simulink model "CS6376_AircraftCollisionAvoidanceProject_RonaldPicard"  (R2018b)
settings: Solver=FixedStepAuto  StartTime=0.0  StopTime=10000  FixedStep=1  RelTol=1e-3
(part 2 of 2)

== stateflow chart CS6376_AircraftCollisionAvoidanceProject_RonaldPicard/Aircraft1/AircraftCollisionAvoidenceController ==
  settings: executeAtInitialization=1  initializeOutput=1
  state Controller
    du:
    Y_Out = Y_State;
    X_Out = X_State;
    Orientation_Out = Orientation_State;
    DangerZoneBreached_Out = 0;
    state CollisionAvoidanceMonitor90
      state InitTurn90_From0
        en:
        Orientation_State = 0;
        X_State = X_State + 1;
        Turning_State = Turning_State - 1;
      state AvoidCollisionTraveling0
        en:
        Orientation_State = 0;
        X_State = X_State + 1;
        Rounds_State = Rounds_State - 1;
        % initialize turn time
        Turning_State = Turning_Rounds_In;
      state InitTurn0
        en:
        Orientation_State = 90;
        Y_State = Y_State + 1;
        Rounds_State = Rounds_In;
        Turning_State = Turning_State - 1;
        % initialize rounds to avoid
        Rounds_State = Rounds_In;
      state Traveling90
        en:
        Orientation_State = 90;
        Y_State = Y_State + 1;
        % initialize turn time
        Turning_State = Turning_Rounds_In;
      state AvoidCollisionTraveling180
        en:
        Orientation_State = 180;
        X_State = X_State - 1;
        Rounds_State = Rounds_State - 1;
        % initialize turn time
        Turning_State = Turning_Rounds_In;
      state InitTurn180
        en:
        Orientation_State = 90;
        Y_State = Y_State + 1;
        Turning_State = Turning_State - 1;
        % initialize rounds to avoid
        Rounds_State = Rounds_In;
      state InitTurn90_From180
        en:
        Orientation_State = 180;
        X_State = X_State - 1;
        Turning_State = Turning_State - 1;
      (junction 582) -> InitTurn90_From0 : %else
      (junction 575) -> (junction 577) [order 2]
      (junction 575) -> InitTurn90_From0 [order 1] : % still turning
          | [Turning_State >0]
      (junction 305) -> (junction 582) [order 2]
      (junction 577) -> Traveling90
      (junction 581) -> (junction 575)
      (junction 305) -> Controller.CollisionAvoidanceMonitor90.AvoidCollisionTraveling0 [order 1] : % incoming aircraft quadrant 3 heading up or right
          | [Mess_Rec_In &&...
          | (X_Mess_In <= X_State) && (Y_Mess_In <= Y_State) &&...
          | (Orientation_Mess_In == 0 || Orientation_Mess_In == 90)]
      (junction 314) -> (junction 305) [order 2]
      InitTurn90_From0 -> (junction 581)
      (default) -> Traveling90
      (junction 314) -> Controller.CollisionAvoidanceMonitor90.AvoidCollisionTraveling0 [order 1] : % incoming aircraft quadrant 2 heading right or down
          | [Mess_Rec_In &&...
          | (X_Mess_In <= X_State) && (Y_Mess_In >= Y_State) &&...
          | (Orientation_Mess_In == 0 || Orientation_Mess_In == 270)]
      (junction 419) -> (junction 314) [order 2]
      (junction 298) -> Traveling90 [order 2] : %else
      (junction 298) -> Controller.CollisionAvoidanceMonitor90.InitTurn0 [order 1] : % incoming aircraft quadrant 3 heading up or right
          | [Mess_Rec_In &&...
          | (X_Mess_In <= X_State) && (Y_Mess_In <= Y_State) &&...
          | (Orientation_Mess_In == 0 || Orientation_Mess_In == 90)]
      (junction 308) -> (junction 298) [order 2]
      (junction 494) -> Controller.CollisionAvoidanceMonitor90.InitTurn0 [order 1] : % still turning
          | [Turning_State >0]
      (junction 494) -> Controller.CollisionAvoidanceMonitor90.AvoidCollisionTraveling0 [order 2]
      (junction 488) -> (junction 494)
      (junction 419) -> Controller.CollisionAvoidanceMonitor90.AvoidCollisionTraveling0 [order 1] : % still avoiding
          | [Rounds_State > 0]
      (junction 296) -> (junction 419)
      (junction 308) -> Controller.CollisionAvoidanceMonitor90.InitTurn0 [order 1] : % incoming aircraft quadrant 2 heading right or down
          | [Mess_Rec_In &&...
          | (X_Mess_In <= X_State) && (Y_Mess_In >= Y_State) &&...
          | (Orientation_Mess_In == 0 || Orientation_Mess_In == 270)]
      (junction 299) -> (junction 308) [order 2]
      Controller.CollisionAvoidanceMonitor90.AvoidCollisionTraveling0 -> (junction 296) : %each round
      Controller.CollisionAvoidanceMonitor90.InitTurn0 -> (junction 488) : %each round
      Controller.CollisionAvoidanceMonitor90.AvoidCollisionTraveling180 -> (junction 316) : %each round
      (junction 316) -> (junction 416)
      (junction 491) -> Controller.CollisionAvoidanceMonitor90.InitTurn180 [order 1] : % still turning
          | [Turning_State >0]
      (junction 491) -> Controller.CollisionAvoidanceMonitor90.AvoidCollisionTraveling180 [order 2]
      (junction 489) -> (junction 491)
      (junction 299) -> Controller.CollisionAvoidanceMonitor90.InitTurn180 [order 1] : % incoming aircraft quadrant 1 heading left or down
          | [Mess_Rec_In &&...
          | (X_Mess_In > X_State) && (Y_Mess_In >= Y_State) &&...
          | (Orientation_Mess_In == 180 || Orientation_Mess_In == 270)]
      (junction 309) -> (junction 299) [order 2]
      (junction 416) -> Controller.CollisionAvoidanceMonitor90.AvoidCollisionTraveling180 [order 1] : % still avoiding
          | [Rounds_State > 0]
      (junction 416) -> (junction 301) [order 2]
      Traveling90 -> (junction 309) : %each round
      (junction 309) -> Controller.CollisionAvoidanceMonitor90.InitTurn180 [order 1] : % incoming aircraft quadrant 4 heading up or left
          | [Mess_Rec_In &&...
          | (X_Mess_In > X_State) &&  (Y_Mess_In <= Y_State) &&...
          | (Orientation_Mess_In == 180 || Orientation_Mess_In == 90)]
      (junction 301) -> Controller.CollisionAvoidanceMonitor90.AvoidCollisionTraveling180 [order 1] : % incoming aircraft quadrant 1 heading left or down
          | [Mess_Rec_In &&...
          | (X_Mess_In > X_State) && (Y_Mess_In >= Y_State) &&...
          | (Orientation_Mess_In == 180 || Orientation_Mess_In == 270)]
      (junction 301) -> (junction 311) [order 2]
      Controller.CollisionAvoidanceMonitor90.InitTurn180 -> (junction 489) : %each round
      (junction 586) -> Traveling90
      (junction 311) -> Controller.CollisionAvoidanceMonitor90.AvoidCollisionTraveling180 [order 1] : % incoming aircraft quadrant 4 heading up or left
          | [Mess_Rec_In &&...
          | (X_Mess_In > X_State) &&  (Y_Mess_In <= Y_State) &&...
          | (Orientation_Mess_In == 180 || Orientation_Mess_In == 90)]
      (junction 311) -> (junction 594) [order 2]
      (junction 588) -> (junction 586) [order 2]
      (junction 588) -> InitTurn90_From180 [order 1] : % still turning
          | [Turning_State >0]
      (junction 587) -> (junction 588)
      (junction 594) -> InitTurn90_From180 : %else
      InitTurn90_From180 -> (junction 587)
    state Turn180_From90
      en:
      Orientation_State = 90;
      Y_State = Y_State + 1;
      Turning_State = Turning_State - 1;
    state Turn90_From0
      en:
      Orientation_State = 0;
      X_State = X_State + 1;
      Turning_State = Turning_State - 1;
    state Turn_90_From180
      en:
      Orientation_State = 180;
      X_State = X_State - 1;
      Turning_State = Turning_State - 1;
    state Turn90_From01
      en:
      Orientation_State = 90;
      Y_State = Y_State + 1;
      Turning_State = Turning_State - 1;
    state CollisionAvoidanceMonitor0
      state Turn0_From90
        en:
        Orientation_State = 90;
        Y_State = Y_State + 1;
        Turning_State = Turning_State - 1;
      state AvoidCollisionTraveling90
        en:
        Orientation_State = 90;
        Y_State = Y_State + 1;
        Rounds_State = Rounds_State - 1;
        % initialize turn time
        Turning_State = Turning_Rounds_In;
      state Turn90
        en:
        Orientation_State = 0;
        X_State = X_State + 1;
        Turning_State = Turning_State - 1;
        % initialize rounds to avoid
        Rounds_State = Rounds_In;
      state Traveling0
        en:
        Orientation_State = 0;
        X_State = X_State + 1;
        % initialize turn time
        Turning_State = Turning_Rounds_In;
      state Turn270
        en:
        Orientation_State = 0;
        X_State = X_State + 1;
        Turning_State = Turning_State - 1;
        % initialize rounds to avoid
        Rounds_State = Rounds_In;
      state AvoidCollisionTraveling270
        en:
        Orientation_State = 270;
        Y_State = Y_State - 1;
        Rounds_State = Rounds_State - 1;
        % initialize turn time
        Turning_State = Turning_Rounds_In;
      state Turn0_From270
        en:
        Orientation_State = 270;
        Y_State = Y_State - 1;
        Turning_State = Turning_State - 1;
      (junction 518) -> Turn0_From90 : %else
      (junction 227) -> (junction 518) [order 2]
      (junction 513) -> (junction 520) [order 2]
      (junction 513) -> Turn0_From90 [order 1] : % still turning
          | [Turning_State >0]
      (junction 520) -> Traveling0
      (junction 516) -> (junction 513)
      Turn0_From90 -> (junction 516)
      (junction 227) -> Controller.CollisionAvoidanceMonitor0.AvoidCollisionTraveling90 [order 1] : % incoming aircraft quadrant 3 heading up or right
          | [Mess_Rec_In &&...
          | (X_Mess_In <= X_State) && (Y_Mess_In <= Y_State) &&...
          | (Orientation_Mess_In == 0 || Orientation_Mess_In == 90)]
      (junction 219) -> (junction 227) [order 2]
      (default) -> Traveling0
      (junction 219) -> Controller.CollisionAvoidanceMonitor0.AvoidCollisionTraveling90 [order 1] : % incoming aircraft quadrant 4 heading up or left
          | [Mess_Rec_In &&...
          | (X_Mess_In >= X_State) && (Y_Mess_In <= Y_State) &&...
          | (Orientation_Mess_In == 180 || Orientation_Mess_In == 90)]
      (junction 381) -> (junction 219) [order 2]
      (junction 450) -> Turn90 [order 1] : % still turning
          | [Turning_State >0]
      (junction 450) -> Controller.CollisionAvoidanceMonitor0.AvoidCollisionTraveling90 [order 2]
      (junction 446) -> (junction 450)
      (junction 207) -> Traveling0 [order 2] : %else
      (junction 207) -> Turn90 [order 1] : % incoming aircraft quadrant 3 heading up or right
          | [Mess_Rec_In &&...
          | (X_Mess_In <= X_State) && (Y_Mess_In <= Y_State) &&...
          | (Orientation_Mess_In == 0 || Orientation_Mess_In == 90)]
      (junction 206) -> (junction 207) [order 2]
      (junction 381) -> Controller.CollisionAvoidanceMonitor0.AvoidCollisionTraveling90 [order 1] : % still avoiding
          | [Rounds_State > 0]
      (junction 220) -> (junction 381)
      Turn90 -> (junction 446) : %each round
      (junction 206) -> Turn90 [order 1] : % incoming aircraft quadrant 4 heading up or left
          | [Mess_Rec_In &&...
          | (X_Mess_In >= X_State) &&  (Y_Mess_In <= Y_State) &&...
          | (Orientation_Mess_In == 180 || Orientation_Mess_In == 90)]
      Controller.CollisionAvoidanceMonitor0.AvoidCollisionTraveling90 -> (junction 220) : %each round
      (junction 213) -> (junction 206) [order 2]
      Controller.CollisionAvoidanceMonitor0.AvoidCollisionTraveling270 -> (junction 230) : %each round
      (junction 213) -> Turn270 [order 1] : % incoming aircraft quadrant 1 heading left or down
          | [Mess_Rec_In &&...
          | (X_Mess_In >= X_State) && (Y_Mess_In > Y_State) &&...
          | (Orientation_Mess_In == 180 || Orientation_Mess_In == 270)]
      (junction 230) -> (junction 384)
      (junction 457) -> Controller.CollisionAvoidanceMonitor0.AvoidCollisionTraveling270 [order 2]
      (junction 457) -> Turn270 [order 1] : % still turning
          | [Turning_State >0]
      (junction 212) -> (junction 213) [order 2]
      (junction 455) -> (junction 457)
      (junction 384) -> Controller.CollisionAvoidanceMonitor0.AvoidCollisionTraveling270 [order 1] : % still avoiding
          | [Rounds_State > 0]
      (junction 384) -> (junction 240) [order 2]
      Traveling0 -> (junction 212) : %each round
      (junction 212) -> Turn270 [order 1] : % incoming aircraft quadrant 2 heading right or down
          | [Mess_Rec_In &&...
          | (X_Mess_In <= X_State) && (Y_Mess_In > Y_State) &&...
          | (Orientation_Mess_In == 0 || Orientation_Mess_In == 270)]
      (junction 240) -> Controller.CollisionAvoidanceMonitor0.AvoidCollisionTraveling270 [order 1] : % incoming aircraft quadrant 1 heading left or down
          | [Mess_Rec_In &&...
          | (X_Mess_In >= X_State) && (Y_Mess_In > Y_State) &&...
          | (Orientation_Mess_In == 180 || Orientation_Mess_In == 270)]
      Turn270 -> (junction 455) : %each round
      (junction 240) -> (junction 238) [order 2]
      (junction 508) -> Traveling0
      (junction 238) -> Controller.CollisionAvoidanceMonitor0.AvoidCollisionTraveling270 [order 1] : % incoming aircraft quadrant 2 heading right or down
          | [Mess_Rec_In &&...
          | (X_Mess_In <= X_State) && (Y_Mess_In > Y_State) &&...
          | (Orientation_Mess_In == 0 || Orientation_Mess_In == 270)]
      (junction 238) -> (junction 498) [order 2]
      (junction 504) -> (junction 508) [order 2]
      (junction 504) -> Controller.CollisionAvoidanceMonitor0.Turn0_From270 [order 1] : % still turning
          | [Turning_State >0]
      (junction 502) -> (junction 504)
      Controller.CollisionAvoidanceMonitor0.Turn0_From270 -> (junction 502)
      (junction 498) -> Controller.CollisionAvoidanceMonitor0.Turn0_From270 : %else
    state CollisionAvoidanceMonitor180
      state InitTurn180_From90
        en:
        Orientation_State = 90;
        Y_State = Y_State + 1;
        Turning_State = Turning_State - 1;
      state AvoidCollisionTraveling90
        en:
        Orientation_State = 90;
        Y_State = Y_State + 1;
        Rounds_State = Rounds_State - 1;
        % initialize turn time
        Turning_State = Turning_Rounds_In;
      state Traveling180
        en:
        Orientation_State = 180;
        X_State = X_State - 1;
        % initialize turn time
        Turning_State = Turning_Rounds_In;
      state InitTurn90
        en:
        Orientation_State = 180;
        X_State = X_State - 1;
        Turning_State = Turning_State - 1;
        % initialize rounds to avoid
        Rounds_State = Rounds_In;
      state AvoidCollisionTraveling270
        en:
        Orientation_State = 270;
        Y_State = Y_State - 1;
        Rounds_State = Rounds_State - 1;
        % initialize turn time
        Turning_State = Turning_Rounds_In;
      state InitTurn270
        en:
        Orientation_State = 180;
        X_State = X_State - 1;
        Turning_State = Turning_State - 1;
        % initialize rounds to avoid
        Rounds_State = Rounds_In;
      state InitTurn180_From270
        en:
        Orientation_State = 270;
        Y_State = Y_State - 1;
        Turning_State = Turning_State - 1;
      (junction 544) -> InitTurn180_From90 : %else
      (junction 286) -> (junction 544) [order 2]
      (junction 538) -> (junction 543) [order 2]
      (junction 538) -> InitTurn180_From90 [order 1] : % still turning
          | [Turning_State >0]
      (junction 543) -> Traveling180
      (junction 540) -> (junction 538)
      (junction 286) -> Controller.CollisionAvoidanceMonitor180.AvoidCollisionTraveling90 [order 1] : % incoming aircraft quadrant 3 heading up or right
          | [Mess_Rec_In &&...
          | (X_Mess_In <= X_State) && (Y_Mess_In < Y_State) &&...
          | (Orientation_Mess_In == 0 || Orientation_Mess_In == 90)]
      InitTurn180_From90 -> (junction 540)
      (junction 269) -> (junction 286) [order 2]
      (default) -> Traveling180
      (junction 269) -> Controller.CollisionAvoidanceMonitor180.AvoidCollisionTraveling90 [order 1] : % incoming aircraft quadrant 4 heading up or left
          | [Mess_Rec_In &&...
          | (X_Mess_In >= X_State) && (Y_Mess_In < Y_State) &&...
          | (Orientation_Mess_In == 180 || Orientation_Mess_In == 90)]
      (junction 406) -> (junction 269) [order 2]
      (junction 279) -> InitTurn90 [order 1] : % incoming aircraft quadrant 3 heading up or right
          | [Mess_Rec_In &&...
          | (X_Mess_In <= X_State) && (Y_Mess_In < Y_State) &&...
          | (Orientation_Mess_In == 0 || Orientation_Mess_In == 90)]
      (junction 279) -> Traveling180 [order 2] : %else
      (junction 483) -> InitTurn90 [order 1] : % still turning
          | [Turning_State >0]
      (junction 483) -> Controller.CollisionAvoidanceMonitor180.AvoidCollisionTraveling90 [order 2]
      (junction 287) -> (junction 279) [order 2]
      (junction 479) -> (junction 483)
      (junction 406) -> Controller.CollisionAvoidanceMonitor180.AvoidCollisionTraveling90 [order 1] : % still avoiding
          | [Rounds_State > 0]
      (junction 288) -> (junction 406)
      (junction 287) -> InitTurn90 [order 1] : % incoming aircraft quadrant 4 heading up or left
          | [Mess_Rec_In &&...
          | (X_Mess_In >= X_State) &&  (Y_Mess_In < Y_State) &&...
          | (Orientation_Mess_In == 180 || Orientation_Mess_In == 90)]
      (junction 276) -> (junction 287) [order 2]
      InitTurn90 -> (junction 479) : %each round
      Controller.CollisionAvoidanceMonitor180.AvoidCollisionTraveling90 -> (junction 288) : %each round
      (junction 481) -> Controller.CollisionAvoidanceMonitor180.AvoidCollisionTraveling270 [order 2]
      (junction 481) -> InitTurn270 [order 1] : % still turning
          | [Turning_State >0]
      (junction 276) -> InitTurn270 [order 1] : % incoming aircraft quadrant 1 heading left or down
          | [Mess_Rec_In &&...
          | (X_Mess_In >= X_State) && (Y_Mess_In >= Y_State) &&...
          | (Orientation_Mess_In == 180 || Orientation_Mess_In == 270)]
      Controller.CollisionAvoidanceMonitor180.AvoidCollisionTraveling270 -> (junction 270) : %each round
      (junction 475) -> (junction 481)
      (junction 271) -> (junction 276) [order 2]
      (junction 270) -> (junction 404)
      Traveling180 -> (junction 271) : %each round
      (junction 271) -> InitTurn270 [order 1] : % incoming aircraft quadrant 2 heading right or down
          | [Mess_Rec_In &&...
          | (X_Mess_In <= X_State) && (Y_Mess_In >= Y_State) &&...
          | (Orientation_Mess_In == 0 || Orientation_Mess_In == 270)]
      (junction 404) -> Controller.CollisionAvoidanceMonitor180.AvoidCollisionTraveling270 [order 1] : % still avoiding
          | [Rounds_State > 0]
      (junction 404) -> (junction 289) [order 2]
      InitTurn270 -> (junction 475) : %each round
      (junction 289) -> Controller.CollisionAvoidanceMonitor180.AvoidCollisionTraveling270 [order 1] : % incoming aircraft quadrant 1 heading left or down
          | [Mess_Rec_In &&...
          | (X_Mess_In >= X_State) && (Y_Mess_In >= Y_State) &&...
          | (Orientation_Mess_In == 180 || Orientation_Mess_In == 270)]
      (junction 289) -> (junction 272) [order 2]
      (junction 526) -> Traveling180
      (junction 272) -> Controller.CollisionAvoidanceMonitor180.AvoidCollisionTraveling270 [order 1] : % incoming aircraft quadrant 2 heading right or down
          | [Mess_Rec_In &&...
          | (X_Mess_In <= X_State) && (Y_Mess_In >= Y_State) &&...
          | (Orientation_Mess_In == 0 || Orientation_Mess_In == 270)]
      (junction 272) -> (junction 532) [order 2]
      (junction 525) -> (junction 526) [order 2]
      (junction 525) -> InitTurn180_From270 [order 1] : % still turning
          | [Turning_State >0]
      (junction 530) -> (junction 525)
      InitTurn180_From270 -> (junction 530)
      (junction 532) -> InitTurn180_From270 : %else
    state Initialize
      en:
      X_State = Initial_X;
      Y_State = Initial_Y;
      Orientation_State = Initial_Orientation;
    state CollisionAvoidanceMonitor270
      state InitTurn270_From0
        en:
        Orientation_State = 0;
        X_State = X_State + 1;
        Turning_State = Turning_State - 1;
      state AvoidCollisionTraveling0
        en:
        Orientation_State = 0;
        X_State = X_State + 1;
        Rounds_State = Rounds_State - 1;
        % initialize turn time
        Turning_State = Turning_Rounds_In;
      state InitTurn0
        en:
        Orientation_State = 270;
        Y_State = Y_State - 1
        Turning_State = Turning_State - 1;
        % initialize rounds to avoid
        Rounds_State = Rounds_In;
      state Traveling270
        en:
        Orientation_State = 270;
        Y_State = Y_State - 1
        % initialize turn time
        Turning_State = Turning_Rounds_In;
      state InitTurn180
        en:
        Orientation_State = 270;
        Y_State = Y_State - 1
        Turning_State = Turning_State - 1;
        % initialize rounds to avoid
        Rounds_State = Rounds_In;
      state AvoidCollisionTraveling180
        en:
        Orientation_State = 180;
        X_State = X_State - 1;
        Rounds_State = Rounds_State - 1;
        % initialize turn time
        Turning_State = Turning_Rounds_In;
      state InitTurn270_From180
        en:
        Orientation_State = 180;
        X_State = X_State - 1;
        Turning_State = Turning_State - 1;
      (junction 569) -> InitTurn270_From0 : %else
      (junction 563) -> (junction 565) [order 2]
      (junction 563) -> InitTurn270_From0 [order 1] : % still turning
          | [Turning_State >0]
      (junction 338) -> (junction 569) [order 2]
      (junction 565) -> Traveling270
      (junction 568) -> (junction 563)
      InitTurn270_From0 -> (junction 568)
      (junction 338) -> Controller.CollisionAvoidanceMonitor270.AvoidCollisionTraveling0 [order 1] : % incoming aircraft quadrant 3 heading up or right
          | [Mess_Rec_In &&...
          | (X_Mess_In < X_State) && (Y_Mess_In <= Y_State) &&...
          | (Orientation_Mess_In == 0 || Orientation_Mess_In == 90)]
      (junction 354) -> (junction 338) [order 2]
      (default) -> Traveling270
      (junction 354) -> Controller.CollisionAvoidanceMonitor270.AvoidCollisionTraveling0 [order 1] : % incoming aircraft quadrant 2 heading right or down
          | [Mess_Rec_In &&...
          | (X_Mess_In < X_State) && (Y_Mess_In >= Y_State) &&...
          | (Orientation_Mess_In == 0 || Orientation_Mess_In == 270)]
      (junction 394) -> (junction 354) [order 2]
      (junction 466) -> Controller.CollisionAvoidanceMonitor270.AvoidCollisionTraveling0 [order 2]
      (junction 466) -> Controller.CollisionAvoidanceMonitor270.InitTurn0 [order 1] : % still turning
          | [Turning_State >0]
      (junction 460) -> (junction 466)
      (junction 333) -> Controller.CollisionAvoidanceMonitor270.InitTurn0 [order 1] : % incoming aircraft quadrant 3 heading up or right
          | [Mess_Rec_In &&...
          | (X_Mess_In < X_State) && (Y_Mess_In <= Y_State) &&...
          | (Orientation_Mess_In == 0 || Orientation_Mess_In == 90)]
      (junction 333) -> Traveling270 [order 2] : %else
      (junction 357) -> (junction 333) [order 2]
      (junction 394) -> Controller.CollisionAvoidanceMonitor270.AvoidCollisionTraveling0 [order 1] : % still avoiding
          | [Rounds_State > 0]
      (junction 337) -> (junction 394)
      (junction 357) -> Controller.CollisionAvoidanceMonitor270.InitTurn0 [order 1] : % incoming aircraft quadrant 2 heading right or down
          | [Mess_Rec_In &&...
          | (X_Mess_In < X_State) && (Y_Mess_In >= Y_State) &&...
          | (Orientation_Mess_In == 0 || Orientation_Mess_In == 270)]
      Controller.CollisionAvoidanceMonitor270.InitTurn0 -> (junction 460) : %each round
      (junction 334) -> (junction 357) [order 2]
      Controller.CollisionAvoidanceMonitor270.AvoidCollisionTraveling0 -> (junction 337) : %each round
      (junction 464) -> Controller.CollisionAvoidanceMonitor270.InitTurn180 [order 1] : % still turning
          | [Turning_State >0]
      (junction 464) -> Controller.CollisionAvoidanceMonitor270.AvoidCollisionTraveling180 [order 2]
      Controller.CollisionAvoidanceMonitor270.AvoidCollisionTraveling180 -> (junction 361) : %each round
      (junction 469) -> (junction 464)
      (junction 361) -> (junction 397)
      (junction 334) -> Controller.CollisionAvoidanceMonitor270.InitTurn180 [order 1] : % incoming aircraft quadrant 1 heading left or down
          | [Mess_Rec_In &&...
          | (X_Mess_In >= X_State) && (Y_Mess_In >= Y_State) &&...
          | (Orientation_Mess_In == 180 || Orientation_Mess_In == 270)]
      (junction 347) -> (junction 334) [order 2]
      (junction 397) -> Controller.CollisionAvoidanceMonitor270.AvoidCollisionTraveling180 [order 1] : % still avoiding
          | [Rounds_State > 0]
      (junction 397) -> (junction 335) [order 2]
      (junction 347) -> Controller.CollisionAvoidanceMonitor270.InitTurn180 [order 1] : % incoming aircraft quadrant 4 heading up or left
          | [Mess_Rec_In &&...
          | (X_Mess_In >= X_State) &&  (Y_Mess_In <= Y_State) &&...
          | (Orientation_Mess_In == 180 || Orientation_Mess_In == 90)]
      Traveling270 -> (junction 347) : %each round
      Controller.CollisionAvoidanceMonitor270.InitTurn180 -> (junction 469) : %each round
      (junction 335) -> Controller.CollisionAvoidanceMonitor270.AvoidCollisionTraveling180 [order 1] : % incoming aircraft quadrant 1 heading left or down
          | [Mess_Rec_In &&...
          | (X_Mess_In >= X_State) && (Y_Mess_In >= Y_State) &&...
          | (Orientation_Mess_In == 180 || Orientation_Mess_In == 270)]
      (junction 551) -> Traveling270
      (junction 335) -> (junction 345) [order 2]
      (junction 345) -> Controller.CollisionAvoidanceMonitor270.AvoidCollisionTraveling180 [order 1] : % incoming aircraft quadrant 4 heading up or left
          | [Mess_Rec_In &&...
          | (X_Mess_In >= X_State) &&  (Y_Mess_In <= Y_State) &&...
          | (Orientation_Mess_In == 180 || Orientation_Mess_In == 90)]
      (junction 345) -> (junction 557) [order 2]
      (junction 549) -> (junction 551) [order 2]
      (junction 549) -> InitTurn270_From180 [order 1] : % still turning
          | [Turning_State >0]
      (junction 556) -> (junction 549)
      InitTurn270_From180 -> (junction 556)
      (junction 557) -> InitTurn270_From180 : %else
    state Turn270_From0
      en:
      Orientation_State = 0;
      X_State = X_State + 1;
      Turning_State = Turning_State - 1;
    state Turn180_From270
      en:
      Orientation_State = 270;
      Y_State = Y_State - 1;
      Turning_State = Turning_State - 1;
    state Turn270_From180
      en:
      Orientation_State = 180;
      X_State = X_State - 1;
      Turning_State = Turning_State - 1;
    state Turn0_From270
      en:
      Orientation_State = 270;
      Y_State = Y_State - 1;
      Turning_State = Turning_State - 1;
    CollisionAvoidanceMonitor90 -> Turn180_From90 [order 2] : [(Y_In<=Y_State+Turning_Rounds_In) && (X_In<X_State)]
    (junction 600) -> CollisionAvoidanceMonitor90 [order 2]
    (junction 600) -> Turn90_From0 [order 1] : % still turning
        | [Turning_State >0]
    (junction 632) -> Turn180_From90 [order 1] : % still turning
        | [Turning_State >0]
    Turn180_From90 -> (junction 631)
    (junction 602) -> (junction 600)
    (junction 636) -> Turn_90_From180 [order 1] : % still turning
        | [Turning_State >0]
    (junction 636) -> CollisionAvoidanceMonitor90 [order 2]
    (junction 631) -> (junction 632)
    (junction 639) -> (junction 636)
    (junction 632) -> CollisionAvoidanceMonitor180 [order 2]
    Turn90_From0 -> (junction 602)
    CollisionAvoidanceMonitor0 -> Turn90_From0 [order 1] : [(X_In<=X_State+Turning_Rounds_In) && (Y_In>=Y_State)]
    Turn_90_From180 -> (junction 639)
    CollisionAvoidanceMonitor180 -> Turn_90_From180 [order 1] : [(X_In>=X_State-Turning_Rounds_In) && (Y_In>=Y_State)]
    CollisionAvoidanceMonitor90 -> Turn90_From01 [order 1] : [(Y_In<=Y_State+Turning_Rounds_In) && (X_In>=X_State)]
    (junction 608) -> Turn90_From01 [order 1] : % still turning
        | [Turning_State >0]
    Turn90_From01 -> (junction 607)
    (junction 607) -> (junction 608)
    (junction 608) -> CollisionAvoidanceMonitor0 [order 2]
    Initialize -> CollisionAvoidanceMonitor90 [order 3] : [Orientation_State == 90]
    (default) -> Initialize
    Initialize -> CollisionAvoidanceMonitor0 [order 1] : [Orientation_State == 0]
    Initialize -> CollisionAvoidanceMonitor180 [order 4] : [Orientation_State == 180]
    Initialize -> CollisionAvoidanceMonitor270 [order 2] : [Orientation_State == 270]
    CollisionAvoidanceMonitor0 -> Turn270_From0 [order 2] : [(X_In<=X_State+Turning_Rounds_In) && (Y_In<Y_State)]
    (junction 623) -> CollisionAvoidanceMonitor0 [order 2]
    CollisionAvoidanceMonitor180 -> Turn270_From180 [order 2] : [(X_In>=X_State-Turning_Rounds_In) && (Y_In<Y_State)]
    (junction 661) -> CollisionAvoidanceMonitor180 [order 2]
    (junction 664) -> (junction 661)
    (junction 661) -> Turn180_From270 [order 1] : % still turning
        | [Turning_State >0]
    Turn180_From270 -> (junction 664)
    (junction 617) -> CollisionAvoidanceMonitor270 [order 2]
    (junction 617) -> Turn270_From0 [order 1] : % still turning
        | [Turning_State >0]
    (junction 616) -> (junction 617)
    Turn270_From0 -> (junction 616)
    CollisionAvoidanceMonitor270 -> Turn180_From270 [order 2] : [(Y_In>=Y_State-Turning_Rounds_In) && (X_In<X_State)]
    (junction 649) -> Turn270_From180 [order 1] : % still turning
        | [Turning_State >0]
    (junction 649) -> CollisionAvoidanceMonitor270 [order 2]
    (junction 652) -> (junction 649)
    Turn270_From180 -> (junction 652)
    (junction 624) -> (junction 623)
    (junction 623) -> Controller.Turn0_From270 [order 1] : % still turning
        | [Turning_State >0]
    Controller.Turn0_From270 -> (junction 624)
    CollisionAvoidanceMonitor270 -> Controller.Turn0_From270 [order 1] : [(Y_In>=Y_State-Turning_Rounds_In) && (X_In>=X_State)]
  state Final
    en, du:
    Y_Out = Y_State;
    X_Out = X_State;
    Orientation_Out = Orientation_State;
    state ErrorDangerZoneBreached
      en, du:
      DangerZoneBreached_Out = 1;
    state DestinationReached
      en, du:
      DangerZoneBreached_Out = 0;
  (default) -> Controller
  Controller -> ErrorDangerZoneBreached [order 1] : % transition to an error state if the danger zone is breached
      | [Mess_Rec_In &&...
      |  X_State - DangerZone_In <  X_Mess_In  &&  X_Mess_In < X_State + DangerZone_In  &&...
      |  Y_State - DangerZone_In <  Y_Mess_In  &&  Y_Mess_In < Y_State + DangerZone_In]
  Controller -> DestinationReached [order 2] : % if final destination is reached
      | [(Y_In==Y_State) && (X_In==X_State)]
  data: Initial_Orientation input; Initial_X input; Initial_Y input; X_In input; Y_In input; X_State local; Y_State local; X_Out output; Y_Out output; X_Mess_In input; Y_Mess_In input; Orientation_Mess_In input; Orientation_State local; Mess_Rec_In input; Orientation_Out output; Rounds_In input; Rounds_State local; DangerZone_In input; DangerZoneBreached_Out output; Turning_Rounds_In input; Turning_State local

== stateflow chart CS6376_AircraftCollisionAvoidanceProject_RonaldPicard/EnviromentCommunications/Enviroment1 ==
  settings: executeAtInitialization=1  initializeOutput=1
  state Environment
    en:
    X_Mess_Out = X_Mess_In;
    Y_Mess_Out = Y_Mess_In;
    Orientation_Mess_Out = Orientation_Mess_In;
  (default) -> Environment
  Environment -> (junction 30) : %each round
  (junction 30) -> (junction 32)
  (junction 32) -> Environment [order 1] : % If aircraft is within the comm zone of the other aircraft
      | [X_In - Comm_Zone_In <=  X_Mess_In  &&  X_Mess_In <= X_In + Comm_Zone_In  &&...
      |  Y_In - Comm_Zone_In <=  Y_Mess_In  &&  Y_Mess_In <= Y_In + Comm_Zone_In]
      | {Send_Mess_Out = 1}
  (junction 32) -> (junction 34) [order 2]
  (junction 34) -> Environment [order 1] : % If aircraft is outside the comm zone of the other aircraft
      | [ X_Mess_In < X_In - Comm_Zone_In  &&  X_In + Comm_Zone_In < X_Mess_In &&...
      |   Y_Mess_In < Y_In - Comm_Zone_In  &&  Y_In + Comm_Zone_In < Y_Mess_In]
      | {Send_Mess_Out = 0}
  (junction 34) -> (junction 41) [order 2]
  (junction 41) -> Environment : %else
  data: Comm_Zone_In input; X_In input; Y_In input; X_Mess_In input; Y_Mess_In input; Orientation_Mess_In input; X_Mess_Out output; Y_Mess_Out output; Orientation_Mess_Out output; Send_Mess_Out output
